simulink model "gm_soc_dvbs2_fpga"  (R2025b)
settings: Solver=VariableStepAuto  StartTime=0.0  StopTime=10.0  RelTol=1e-3
InitFcn:
  | soc_dvbs2_init;
undefined symbols (not defined in the file or in its folder): Add, coefficientsLog, coefficientsSqrt1, coefficientsSqrt2, dataBits, Deinterleaver, designMultirateFIR, noisePow, Shift, Short, soc_dvbs2_designFIRFilter, soc_dvbs2_txPacketBits, syncWord, txDataOut, txFiltCoeff, XData
libraries: simulink x304, hdlsllib x265, dspsigops x15, dsphdlfiltering2 x8, hdlmdlgenlib x6, dsphdlsigops2 x5, commseqgen3 x5, dsphdlmathfun2 x3, hwlogicconnlib x2, whdledac x2, commhdlcrc x2, whdlutilities x1
(part 23 of 36)

== system gm_soc_dvbs2_fpga/DVBS2/DVBS2 TxRx/DVB-S2 HDL Receiver/Synchronizer and PL Header Decoder/Time Frequency and Coarse Phase Synchronizer/Coarse Phase Synchronizer/Coarse Phase Estimator ==
  dataIn : Inport  OutDataTypeStr=fixdt(1, 18, 13)  PortDimensions=1  SampleTime=2.5e-07
      settings: SignalType=complex
  pilotIdx : Inport  Port=2  OutDataTypeStr=fixdt(0, 11, 0)  PortDimensions=1  SampleTime=2.5e-07
  pilotValid : Inport  Port=3  OutDataTypeStr=boolean  PortDimensions=1  SampleTime=2.5e-07
  Add3 : Sum  OutDataTypeStr=fixdt(1, 17, 14)  AccumDataTypeStr=fixdt(1, 18, 14)  SampleTime=2.5e-07
  Compare To Constant1 : simulink/Logic and Bit Operations/Compare To Constant  relop===  const="fi(0,0,11,0,\"hex\",\"5c3\")"  OutDataTypeStr=boolean
  Compare To Constant2 : simulink/Logic and Bit Operations/Compare To Constant  relop===  const="fi(0,0,11,0,\"hex\",\"5a0\")"  OutDataTypeStr=boolean
  Data Type Conversion : DataTypeConversion  OutDataTypeStr=fixdt(1, 17, 14)  SampleTime=2.5e-07  SaturateOnIntegerOverflow=off  RndMeth=Floor
  Delay{,1,8..11,15..17} (9 alike) : Delay  DelayLength=double(1)  InitialCondition=0  SampleTime=2.5e-07
  Delay{2..7,12..14,20} (10 alike) : Delay  DelayLength=double(2)  InitialCondition=0  SampleTime=2.5e-07
  Gain : Gain  Gain="fi(0,1,18,17,\"hex\",\"16a0a + 295f6 i\")"  ParamDataTypeStr=fixdt(1, 18, 17)  OutDataTypeStr=fixdt(1, 18, 13)  SampleTime=2.5e-07
  Gain1 : Gain  Gain="fi(0,0,5,5,\"hex\",\"01\")"  ParamDataTypeStr=fixdt(0, 5, 5)  OutDataTypeStr=fixdt(1, 18, 13)  SampleTime=2.5e-07
  Logical Operator : Logic  AllPortsSameDT=off  OutDataTypeStr=boolean  SampleTime=2.5e-07
  Logical Operator1 : Logic  AllPortsSameDT=off  OutDataTypeStr=boolean  SampleTime=2.5e-07
  Unit Delay Enabled Resettable Synchronous : hdlsllib/Discrete/Unit Delay Enabled Resettable Synchronous  InitialCondition=double(0)  SampleTime=-1
  estimate : Outport  SampleTime=2.5e-07
  estValid : Outport  Port=2  SampleTime=2.5e-07
  wires:
  Delay10/1 -> Unit Delay Enabled Resettable Synchronous/3
  pilotValid/1 -> Delay5/1, Delay16/1, Delay/1
  Delay/1 -> Delay7/1
  dataIn/1 -> Delay1/1
  Delay15/1 -> Compare To Constant1/1
  pilotIdx/1 -> Delay15/1, Compare To Constant2/1
  Delay1/1 -> Delay4/1
  Compare To Constant2/1 -> Delay6/1
  Compare To Constant1/1 -> Delay14/1
  Delay4/1 -> Gain/1
  Delay16/1 -> Delay13/1
  Delay6/1 -> Logical Operator/1
  Delay5/1 -> Logical Operator/2
  Gain/1 -> Delay2/1
  Delay14/1 -> Logical Operator1/1
  Delay13/1 -> Logical Operator1/2
  Delay7/1 -> Delay3/1
  Logical Operator/1 -> Delay20/1
  Delay2/1 -> Gain1/1
  Logical Operator1/1 -> Delay12/1
  Delay3/1 -> Delay9/1
  Delay20/1 -> Delay10/1
  Gain1/1 -> Data Type Conversion/1
  Delay12/1 -> Delay11/1
  Delay9/1 -> Unit Delay Enabled Resettable Synchronous/2
  Data Type Conversion/1 -> Delay8/1
  Delay11/1 -> Delay17/1
  Unit Delay Enabled Resettable Synchronous/1 -> estimate/1, Add3/1
  Delay8/1 -> Add3/2
  Delay17/1 -> estValid/1
  Add3/1 -> Unit Delay Enabled Resettable Synchronous/1

== system gm_soc_dvbs2_fpga/DVBS2/DVBS2 TxRx/DVB-S2 HDL Receiver/Synchronizer and PL Header Decoder/Time Frequency and Coarse Phase Synchronizer/Coarse Phase Synchronizer/Unwrapping algorithm ==
  u : Inport  OutDataTypeStr=fixdt(1, 17, 14)  PortDimensions=1  SampleTime=2.5e-07
      settings: SignalType=complex
  E : Inport  Port=2  OutDataTypeStr=boolean  PortDimensions=1  SampleTime=2.5e-07
  Add : Sum  Inputs=+-  OutDataTypeStr=fixdt(1, 20, 19)  AccumDataTypeStr=fixdt(1, 26, 20)  SampleTime=2.5e-07
  Add1 : Sum  OutDataTypeStr=fixdt(1, 25, 20)  AccumDataTypeStr=fixdt(1, 26, 20)  SampleTime=2.5e-07
  Complex to Magnitude-Angle HDL Optimized : dsphdlmathfun2/Complex to Magnitude-Angle  NumIterationsSource=Auto  NumIterations=10  OutputFormat=Angle  AngleFormat=Normalized  ScaleOutput=on  ScalingMethod=Shift-Add  SimulateUsing=Code generation
  Constant : Constant  OutDataTypeStr=boolean  SampleTime=2.5e-07
  Data Type Conversion : DataTypeConversion  OutDataTypeStr=fixdt(1, 25, 20)  SampleTime=2.5e-07  SaturateOnIntegerOverflow=off  RndMeth=Floor
  Data Type Conversion1 : DataTypeConversion  OutDataTypeStr=fixdt(1, 21, 21)  SampleTime=2.5e-07  SaturateOnIntegerOverflow=off  RndMeth=Floor
  Data Type Conversion2 : DataTypeConversion  OutDataTypeStr=fixdt(1, 21, 0)  ConvertRealWorld=Stored Integer (SI)  SampleTime=2.5e-07  SaturateOnIntegerOverflow=off  RndMeth=Floor
  Gain1 : Gain  Gain="fi(0,0,1,1,\"hex\",\"1\")"  ParamDataTypeStr=fixdt(0, 1, 1)  OutDataTypeStr=fixdt(1, 26, 21)  SampleTime=2.5e-07
  NCO HDL Optimized : dsphdlsigops2/NCO  PhaseIncrementSource=Property  PhaseIncrement=0  PhaseOffsetSource=Input port  PhaseOffset=0  DitherSource=None  NumDitherBits=4  SamplesPerFrame=1  LUTCompress=off  ResetAction=off  Waveform=Complex exponential  PhasePort=off  SimulateUsing=Code generation  AccumulatorWL=21  PhaseQuantization=on  NumQuantizerAccumulatorBits=14  OutputDataType=Binary point scaling  OutputWL=16  OutputFL=14
  NCO HDL Optimized_term1 : Terminator
  PrevEst : hdlsllib/Discrete/Unit Delay Enabled Synchronous  InitialCondition=double(0)  SampleTime=-1
  currentEst : hdlsllib/Discrete/Unit Delay Enabled Synchronous  InitialCondition=double(0)  SampleTime=-1
  estimate : Outport  SampleTime=2.5e-07  VectorParamsAs1DForOutWhenUnconnected=off
  wires:
  u/1 -> Complex to Magnitude-Angle HDL Optimized/1
  E/1 -> Complex to Magnitude-Angle HDL Optimized/2
  Complex to Magnitude-Angle HDL Optimized/1 -> currentEst/1
  Data Type Conversion1/1 -> Data Type Conversion2/1
  currentEst/1 -> Add/1
  Complex to Magnitude-Angle HDL Optimized/2 -> PrevEst/2, currentEst/2
  Data Type Conversion/1 -> Add1/1
  PrevEst/1 -> Add1/2, Add/2
  Add/1 -> Data Type Conversion/1
  Add1/1 -> Gain1/1, PrevEst/1
  Gain1/1 -> Data Type Conversion1/1
  Data Type Conversion2/1 -> NCO HDL Optimized/1
  Constant/1 -> NCO HDL Optimized/2
  NCO HDL Optimized/1 -> estimate/1
  NCO HDL Optimized/2 -> NCO HDL Optimized_term1/1

== system gm_soc_dvbs2_fpga/DVBS2/DVBS2 TxRx/DVB-S2 HDL Receiver/Synchronizer and PL Header Decoder/Time Frequency and Coarse Phase Synchronizer/Fine Frequency Synchronizer/Modified L and R Algorithm ==
  z : Inport  OutDataTypeStr=fixdt(1, 18, 13)  PortDimensions=1  SampleTime=2.5e-07
      settings: SignalType=complex
  zvalid : Inport  Port=2  OutDataTypeStr=boolean  PortDimensions=1  SampleTime=2.5e-07
  pilotIdx : Inport  Port=3  OutDataTypeStr=fixdt(0, 11, 0)  PortDimensions=1  SampleTime=2.5e-07
  Compare To Constant2 : simulink/Logic and Bit Operations/Compare To Constant  relop===  const=config.PilotMaxIdx  OutDataTypeStr=boolean
  Complex to Magnitude-Angle HDL Optimized : dsphdlmathfun2/Complex to Magnitude-Angle  NumIterationsSource=Auto  NumIterations=10  OutputFormat=Angle  AngleFormat=Normalized  ScaleOutput=on  ScalingMethod=Shift-Add  SimulateUsing=Code generation
  Data Type Conversion : DataTypeConversion  OutDataTypeStr=fixdt(1,21,21)  SaturateOnIntegerOverflow=off  RndMeth=Floor
  Data Type Conversion1 : DataTypeConversion  OutDataTypeStr=fixdt(1,43,26)  SaturateOnIntegerOverflow=off  RndMeth=Floor
  Data Type Conversion3 : DataTypeConversion  OutDataTypeStr=fixdt(1,43,40)  ConvertRealWorld=Stored Integer (SI)  SaturateOnIntegerOverflow=off  RndMeth=Floor
  Delay : Delay
  Delay1 : Delay
  Delay2 : Delay
  Delay3 : Delay  DelayLength=28
  Delay4 : Delay  DelayLength=1
  Gain : Gain  Gain=fi(1/19,0,16,16)  ParamDataTypeStr=Inherit: Inherit from 'Gain'  OutDataTypeStr=fixdt(1, 46, 45)
  L and R Algorithm 18 point : Subsystem
  Logical Operator : Logic  AllPortsSameDT=off  OutDataTypeStr=boolean
  Moving Average : Subsystem
  Unit Delay Enabled Synchronous : hdlsllib/Discrete/Unit Delay Enabled Synchronous  InitialCondition=0.0  SampleTime=-1
  estOut : Outport  SampleTime=2.5e-07
  wires:
  Compare To Constant2/1 -> Logical Operator/2
  Logical Operator/1 -> Delay3/1
  L and R Algorithm 18 point/1(dataIn) -> Moving Average/1(dataIn)
  z/1 -> L and R Algorithm 18 point/1(z)
  Complex to Magnitude-Angle HDL Optimized/1 -> Unit Delay Enabled Synchronous/1
  pilotIdx/1 -> Compare To Constant2/1
  Unit Delay Enabled Synchronous/1 -> Delay4/1
  zvalid/1 -> Logical Operator/1, L and R Algorithm 18 point/2(zvalid)
  Delay3/1 -> Delay/1
  Delay/1 -> Moving Average/2(validIn)
  Moving Average/1(dataOut) -> Data Type Conversion1/1
  Moving Average/2(validOut) -> Complex to Magnitude-Angle HDL Optimized/2
  Data Type Conversion1/1 -> Data Type Conversion3/1
  Data Type Conversion3/1 -> Complex to Magnitude-Angle HDL Optimized/1
  Complex to Magnitude-Angle HDL Optimized/2 -> Unit Delay Enabled Synchronous/2
  Delay4/1 -> Delay1/1
  Delay1/1 -> Gain/1
  Gain/1 -> Delay2/1
  Delay2/1 -> Data Type Conversion/1
  Data Type Conversion/1 -> estOut/1

== system gm_soc_dvbs2_fpga/DVBS2/DVBS2 TxRx/DVB-S2 HDL Receiver/Synchronizer and PL Header Decoder/Time Frequency and Coarse Phase Synchronizer/Fine Gain Control/Reciprocal ==
  dataIn : Inport  OutDataTypeStr=fixdt(1, 13, 10)  PortDimensions=1  SampleTime=2.5e-07
  Compare To Constant : simulink/Logic and Bit Operations/Compare To Constant  relop=<  const=0  OutDataTypeStr=boolean
  Compare To Constant1 : simulink/Logic and Bit Operations/Compare To Constant  relop===  const=0  OutDataTypeStr=boolean
  Constant : Constant  OutDataTypeStr=fixdt(1, 26, 14)  SampleTime=-1
  Data Type Conversion : DataTypeConversion  OutDataTypeStr=fixdt(1,WL,0)  ConvertRealWorld=Stored Integer (SI)  SaturateOnIntegerOverflow=off  RndMeth=Floor
  Data Type Conversion1 : DataTypeConversion  OutDataTypeStr=fixdt(0,LUTAddrWL,0)  ConvertRealWorld=Stored Integer (SI)  SaturateOnIntegerOverflow=off  RndMeth=Floor
      mask init:
      | Simulink.suppressDiagnostic(gcb, 'SimulinkFixedPoint:util:Overflowoccurred');
  Data Type Conversion2 : DataTypeConversion  OutDataTypeStr=fixdt(0,WL-LUTAddrWL,0)  ConvertRealWorld=Stored Integer (SI)  SaturateOnIntegerOverflow=off  RndMeth=Floor
  Delay : Delay  DelayLength=1
  Delay1 : Delay  DelayLength=1
  Delay2 : Delay  DelayLength=1
  Delay3 : Delay  DelayLength=7
  Extract Bits : simulink/Logic and Bit Operations/Extract Bits  bitsToExtract=Range ending with least significant bit  numBits=LUTAddrWL  bitIdxRange=[0 7]  outScalingMode=Treat bit field as an integer
  Function Impl : Subsystem
  Switch : Switch  Criteria=u2 > Threshold  OutDataTypeStr=fixdt(1, 26, 14)  SaturateOnIntegerOverflow=off  InputSameDT=off
  dataOut : Outport  SampleTime=2.5e-07
  wires:
  dataIn/1 -> Data Type Conversion/1, Delay3/1
  Delay1/1 -> Data Type Conversion2/1
  Delay3/1 -> Compare To Constant1/1
  Compare To Constant1/1 -> Switch/2
  Data Type Conversion/1 -> Delay/1
  Compare To Constant/1 -> Delay1/1
  Delay/1 -> Extract Bits/1, Compare To Constant/1
  Extract Bits/1 -> Delay2/1
  Delay2/1 -> Data Type Conversion1/1
  Data Type Conversion2/1 -> Function Impl/1(switch)
  Data Type Conversion1/1 -> Function Impl/2(LUTAddr)
  Constant/1 -> Switch/1
  Function Impl/1(functionValues) -> Switch/3
  Switch/1 -> dataOut/1

== system gm_soc_dvbs2_fpga/DVBS2/DVBS2 TxRx/DVB-S2 HDL Receiver/Synchronizer and PL Header Decoder/Time Frequency and Coarse Phase Synchronizer/Time and Coarse Frequency Synchronizer/Coarse Frequency Estimator ==
  rst : Inport  OutDataTypeStr=boolean  PortDimensions=1  SampleTime=2.5e-07
  dataIn : Inport  Port=2  OutDataTypeStr=fixdt(1, 18, 13)  PortDimensions=1  SampleTime=2.5e-07
      settings: SignalType=complex
  pilotValid : Inport  Port=3  OutDataTypeStr=boolean  PortDimensions=1  SampleTime=2.5e-07
  pilotIdx : Inport  Port=4  OutDataTypeStr=fixdt(0, 11, 0)  PortDimensions=1  SampleTime=2.5e-07
  Compare To Constant : simulink/Logic and Bit Operations/Compare To Constant  relop=>  const="fi(0,0,16,0,\"hex\",\"0020\")"  OutDataTypeStr=boolean
  Constant : Constant  Value=0  OutDataTypeStr=boolean  SampleTime=6.25e-08
  Delay : Delay  DelayLength=double(1)  InitialCondition=1  SampleTime=6.25e-08
  Delay{1..4,28} (5 alike) : Delay  DelayLength=double(1)  InitialCondition=0  SampleTime=2.5e-07
  Direct Digital Synthesis : Subsystem
  Frequency Error Detector : Subsystem
  Logical Operator : Logic  Operator=NOT  Inputs=1  AllPortsSameDT=off  OutDataTypeStr=boolean  SampleTime=2.5e-07
  Loop Filter : Subsystem
  Multiport Switch : MultiPortSwitch  DataPortOrder=Zero-based contiguous  Inputs=2  DiagnosticForDefault=None  zeroidx=on  OutDataTypeStr=fixdt(1, 16, 14)  SampleTime=6.25e-08  SaturateOnIntegerOverflow=off  InputSameDT=off
  Pilot Blks Counter : Subsystem
  Unit Delay Enabled Resettable Synchronous : hdlsllib/Discrete/Unit Delay Enabled Resettable Synchronous  InitialCondition=double(0)  SampleTime=-1
  complexEstimate : Outport  SampleTime=6.25e-08
  normFreqEst : Outport  Port=2  SampleTime=2.5e-07
  wires:
  pilotIdx/1 -> Pilot Blks Counter/1(pilotIdx), Frequency Error Detector/2(pilotIdx)
  dataIn/1 -> Frequency Error Detector/1(dataIn)
  Delay2/1 -> Loop Filter/2(rst)
  rst/1 -> Unit Delay Enabled Resettable Synchronous/3, Delay2/1, Pilot Blks Counter/3(rst)
  pilotValid/1 -> Frequency Error Detector/3(pilotValid), Pilot Blks Counter/2(pilotValid)
  Pilot Blks Counter/1(pilotBlkCount) -> Compare To Constant/1
  Frequency Error Detector/1(e) -> Delay28/1
  Compare To Constant/1 -> Unit Delay Enabled Resettable Synchronous/2, Unit Delay Enabled Resettable Synchronous/1
  Delay28/1 -> Loop Filter/1(e)
  Loop Filter/2(rstOut) -> Delay4/1
  Unit Delay Enabled Resettable Synchronous/1 -> Logical Operator/1
  Logical Operator/1 -> Delay1/1
  Delay1/1 -> Loop Filter/3(En)
  Loop Filter/1(v) -> Delay3/1
  Delay3/1 -> Direct Digital Synthesis/1(v)
  Delay4/1 -> Direct Digital Synthesis/2(rst)
  Constant/1 -> Multiport Switch/1
  Direct Digital Synthesis/1(complexEst) -> Multiport Switch/3
  Direct Digital Synthesis/2(normalizedEst) -> normFreqEst/1
  Multiport Switch/1 -> complexEstimate/1, Delay/1
  Delay/1 -> Multiport Switch/2

== system gm_soc_dvbs2_fpga/DVBS2/DVBS2 TxRx/DVB-S2 HDL Receiver/Synchronizer and PL Header Decoder/Time Frequency and Coarse Phase Synchronizer/Time and Coarse Frequency Synchronizer/Frame Synchronizer ==
  dataIn : Inport  OutDataTypeStr=fixdt(1, 18, 13)  PortDimensions=1  SampleTime=2.5e-07
      settings: SignalType=complex
  validIn : Inport  Port=2  OutDataTypeStr=boolean  PortDimensions=1  SampleTime=2.5e-07
  Correlator : Subsystem
  Data Type Conversion : DataTypeConversion  OutDataTypeStr=fixdt(1,15,12)  SaturateOnIntegerOverflow=off  RndMeth=Floor
  Data Type Conversion1 : DataTypeConversion  OutDataTypeStr=fixdt(1,15,11)  SaturateOnIntegerOverflow=off  RndMeth=Floor
  Data Type Conversion2 : DataTypeConversion  OutDataTypeStr=fixdt(1,15,12)  SaturateOnIntegerOverflow=off  RndMeth=Floor
  Delay1 : Delay  DelayLength=70
  Delay{6,9..11} (4 alike) : Delay  DelayLength=9
  Delay12 : Delay
  Delay13 : Delay
  Delay2 : Delay  DelayLength=70
  Delay3 : Delay  DelayLength=config.PLSCLength
  Delay4 : Delay  DelayLength=config.PLSCLength
  Delay5 : Delay  DelayLength=config.PLSCLength
  Pilot and Sync Pulse Indicator : Subsystem
  dataOut : Outport  SampleTime=2.5e-07
  validOut : Outport  Port=2  SampleTime=2.5e-07
  endOfSOF : Outport  Port=3  SampleTime=2.5e-07
  hasPilots : Outport  Port=4  SampleTime=2.5e-07
  VisualizeCorrelationSignals : Outport  Port=5
  wires:
  Pilot and Sync Pulse Indicator/1(hasPilots) -> hasPilots/1
  Delay6/1 -> Delay1/1
  Data Type Conversion/1 -> Pilot and Sync Pulse Indicator/1(SOFCorrDelayed)
  dataIn/1 -> Delay12/1
  validIn/1 -> Delay13/1
  Delay12/1 -> Delay6/1, Correlator/1(dataIn)
  Delay13/1 -> Delay11/1, Correlator/2(validIn)
  Correlator/1(SOFCorrOut) -> Delay5/1
  Correlator/2(PLSCCorrOut) -> Data Type Conversion1/1
  Correlator/3(threshold) -> Data Type Conversion2/1
  Delay11/1 -> Delay2/1
  Delay1/1 -> Delay3/1
  Delay5/1 -> Data Type Conversion/1
  Data Type Conversion2/1 -> Pilot and Sync Pulse Indicator/3(threshold)
  Delay2/1 -> Delay4/1
  Delay3/1 -> Delay10/1
  Data Type Conversion1/1 -> Pilot and Sync Pulse Indicator/2(PLSCCorr)
  Delay4/1 -> Delay9/1
  Delay10/1 -> dataOut/1
  Pilot and Sync Pulse Indicator/2(thresholdExceeded) -> endOfSOF/1
  Pilot and Sync Pulse Indicator/3(VisualizeCorrelationSignals) -> VisualizeCorrelationSignals/1
  Delay9/1 -> validOut/1

== system gm_soc_dvbs2_fpga/DVBS2/DVBS2 TxRx/DVB-S2 HDL Receiver/Synchronizer and PL Header Decoder/Time Frequency and Coarse Phase Synchronizer/Time and Coarse Frequency Synchronizer/PL Data Descrambler and Pilot Valid Indicator ==
  dataIn : Inport  OutDataTypeStr=fixdt(1, 18, 13)  PortDimensions=1  SampleTime=2.5e-07
      settings: SignalType=complex
  validIn : Inport  Port=2  OutDataTypeStr=boolean  PortDimensions=1  SampleTime=2.5e-07
  endOfSOFIn : Inport  Port=3  OutDataTypeStr=boolean  PortDimensions=1  SampleTime=2.5e-07
  hasPilots : Inport  Port=4  OutDataTypeStr=boolean  PortDimensions=1  SampleTime=2.5e-07
  Compare To Constant1 : simulink/Logic and Bit Operations/Compare To Constant  relop===  const=config.PLSCLength - 1  OutDataTypeStr=boolean
  Delay : Delay  DelayLength=config.SOFLength
  Delay1 : Delay  DelayLength=config.SOFLength
  Delay{2..18} (17 alike) : Delay  DelayLength=1
  Delay{19..22} (4 alike) : Delay  DelayLength=14
  Delay23 : Delay  DelayLength=4
  Delay24 : Delay  DelayLength=4
  Input Sample Counter : hdlsllib/Sources/HDL Counter  CountType=Free running  CountInit=0  CountStep=1  CountMax=25  CountFromType=Initial value  CountFrom=0  CountResetPort=on  CountLoadPort=off  CountEnbPort=on  CountDirPort=off  CountHitOutputPort=off  CountDataType=Unsigned  CountWordLen=32  CountFracLen=0  CountSampTime=1
  Logical Operator : Logic  AllPortsSameDT=off  OutDataTypeStr=boolean
  PL Data Descrambler : Subsystem
  Pilot Valid Indicator : Subsystem
  pilotidx : Outport  SampleTime=2.5e-07
  pilotValid : Outport  Port=2  SampleTime=2.5e-07
  dataOut : Outport  Port=3  SampleTime=2.5e-07
  validOut : Outport  Port=4  SampleTime=2.5e-07
  endOfSOF : Outport  Port=5  SampleTime=2.5e-07
  wires:
  endOfSOFIn/1 -> Delay2/1
  validIn/1 -> Delay9/1
  Delay2/1 -> Delay5/1, Input Sample Counter/1
  Delay9/1 -> Input Sample Counter/2, Delay7/1
  hasPilots/1 -> Delay3/1
  Input Sample Counter/1 -> Delay6/1
  Delay7/1 -> Delay12/1, [validIn]
  Delay5/1 -> Delay16/1
  Delay6/1 -> Delay13/1, Compare To Constant1/1
  dataIn/1 -> Delay10/1
  Delay3/1 -> Delay4/1
  Delay/1 -> Delay23/1
  Delay16/1 -> Delay20/1
  [validIn] -> Delay15/1
  Compare To Constant1/1 -> Delay14/1
  Delay10/1 -> Delay8/1
  Delay4/1 -> Delay18/1
  [validIn] -> Delay17/1
  PL Data Descrambler/1(dataOut) -> Delay/1
  Delay15/1 -> Logical Operator/1
  Pilot Valid Indicator/2(pilotIdx) -> pilotidx/1
  Delay14/1 -> Logical Operator/2
  Delay20/1 -> Pilot Valid Indicator/3(endOfSOFIn)
  Delay13/1 -> PL Data Descrambler/2(inputCount)
  Delay8/1 -> Delay11/1
  Delay18/1 -> Delay22/1
  Delay1/1 -> Delay24/1
  Delay17/1 -> Delay21/1
  Logical Operator/1 -> Delay19/1, PL Data Descrambler/1(reset)
  Delay12/1 -> PL Data Descrambler/3(validIn)
  Pilot Valid Indicator/1(pilotValid) -> pilotValid/1
  Delay11/1 -> PL Data Descrambler/4(dataIn)
  Delay22/1 -> Pilot Valid Indicator/1(pilotEnable)
  Delay21/1 -> Pilot Valid Indicator/2(validIn)
  Delay19/1 -> Pilot Valid Indicator/4(endOfPLSC)
  PL Data Descrambler/2(validOut) -> Delay1/1
  Pilot Valid Indicator/3(endOfSOF) -> endOfSOF/1
  Delay23/1 -> dataOut/1
  Delay24/1 -> validOut/1

== system gm_soc_dvbs2_fpga/DVBS2/DVBS2 TxRx/DVB-S2 HDL Receiver/Synchronizer and PL Header Decoder/Time Frequency and Coarse Phase Synchronizer/Time and Coarse Frequency Synchronizer/Symbol Synchronizer ==
  dataIn : Inport  OutDataTypeStr=fixdt(1, 18, 13)  PortDimensions=1  SampleTime=6.25e-08
      settings: SignalType=complex
  validIn : Inport  Port=2  OutDataTypeStr=boolean  PortDimensions=1  SampleTime=6.25e-08
  Data Type Conversion : DataTypeConversion  OutDataTypeStr=fixdt(1, 18, 13)  SampleTime=6.25e-08  SaturateOnIntegerOverflow=off  RndMeth=Floor
  Delay{1..4,6,8..9} (7 alike) : Delay  DelayLength=double(1)  InitialCondition=0  SampleTime=6.25e-08
  Delay5 : Delay  DelayLength=double(12)  InitialCondition=0  SampleTime=6.25e-08
  Delay7 : Delay  DelayLength=double(12)  InitialCondition=0  SampleTime=6.25e-08
  Gardner TED : Subsystem
  Integer Delay{1..4} (4 alike) : Delay  DelayLength=double(1)  InitialCondition=0  SampleTime=6.25e-08
  Interpolation Control : Subsystem
  Interpolation Filter : Subsystem
  Loop Filter : Subsystem
  Rate Handle : Subsystem
  dataOut : Outport  SampleTime=2.5e-07
  validOut : Outport  Port=2  SampleTime=2.5e-07
  wires:
  Loop Filter/1(v) -> Delay4/1
  Interpolation Control/2(Underflow) -> Integer Delay3/1
  Delay4/1 -> Interpolation Control/1(Delta)
  dataIn/1 -> Integer Delay1/1
  Delay5/1 -> Delay2/1, Delay9/1
  Interpolation Control/1(mu) -> Integer Delay4/1
  Integer Delay3/1 -> Delay5/1
  Integer Delay4/1 -> Interpolation Filter/2(mu)
  Gardner TED/1(e) -> Delay3/1
  Integer Delay1/1 -> Interpolation Filter/1(In)
  validIn/1 -> Integer Delay2/1
  Delay1/1 -> Rate Handle/1(dataIn)
  Interpolation Filter/1(interpolant) -> Delay8/1, Data Type Conversion/1
  Integer Delay2/1 -> Delay7/1
  Delay8/1 -> Gardner TED/1(data)
  Delay9/1 -> Gardner TED/2(strobe)
  Data Type Conversion/1 -> Delay1/1
  Delay7/1 -> Delay6/1
  Delay2/1 -> Rate Handle/2(strobe)
  Delay6/1 -> Rate Handle/3(validIn)
  Delay3/1 -> Loop Filter/1(e)
  Rate Handle/1(dataOut) -> dataOut/1
  Rate Handle/2(validOut) -> validOut/1

== system gm_soc_dvbs2_fpga/DVBS2/DVBS2 TxRx/LUT Based Tx/Subsystem1/Subsystem/txLUT1/1-D Lookup Table ==
  In1 : Inport
  1-D Lookup Table : Lookup_n-D  NumberOfTableDimensions=1  BreakpointsSpecification=Even spacing  BreakpointsForDimension1=0:length(txDataOut)-1  BreakpointsForDimension1FirstPoint=0  Table=fi(DataLUT,1,18,16)  TableDataTypeStr=Inherit: Inherit from 'Table data'  InterpMethod=Flat  InternalRulePriority=Speed  OutDataTypeStr=fixdt(1, 18, 16)  RndMeth=Simplest
  1-D Lookup Table_pd1 : Delay  DelayLength=1
  Out1 : Outport
  wires:
  In1/1 -> 1-D Lookup Table/1
  1-D Lookup Table_pd1/1 -> Out1/1
  1-D Lookup Table/1 -> 1-D Lookup Table_pd1/1

== system gm_soc_dvbs2_fpga/DVBS2/DVBS2 TxRx/LUT Based Tx/Subsystem1/Subsystem/txLUT2/1-D Lookup Table ==
  In1 : Inport
  1-D Lookup Table : Lookup_n-D  NumberOfTableDimensions=1  BreakpointsSpecification=Even spacing  BreakpointsForDimension1=0:length(txDataOut)-1  BreakpointsForDimension1FirstPoint=0  Table=fi(DataLUT,1,18,16)  TableDataTypeStr=Inherit: Inherit from 'Table data'  InterpMethod=Flat  InternalRulePriority=Speed  OutDataTypeStr=fixdt(1, 18, 16)  RndMeth=Simplest
  1-D Lookup Table_pd1 : Delay  DelayLength=1
  Out1 : Outport
  wires:
  In1/1 -> 1-D Lookup Table/1
  1-D Lookup Table_pd1/1 -> Out1/1
  1-D Lookup Table/1 -> 1-D Lookup Table_pd1/1

== system gm_soc_dvbs2_fpga/DVBS2/DVBS2 TxRx/LUT Based Tx/Subsystem1/Subsystem/txLUT3/1-D Lookup Table ==
  In1 : Inport
  1-D Lookup Table : Lookup_n-D  NumberOfTableDimensions=1  BreakpointsSpecification=Even spacing  BreakpointsForDimension1=0:length(txDataOut)-1  BreakpointsForDimension1FirstPoint=0  Table=fi(DataLUT,1,18,16)  TableDataTypeStr=Inherit: Inherit from 'Table data'  InterpMethod=Flat  InternalRulePriority=Speed  OutDataTypeStr=fixdt(1, 18, 16)  RndMeth=Simplest
  1-D Lookup Table_pd1 : Delay  DelayLength=1
  Out1 : Outport
  wires:
  In1/1 -> 1-D Lookup Table/1
  1-D Lookup Table_pd1/1 -> Out1/1
  1-D Lookup Table/1 -> 1-D Lookup Table_pd1/1

== system gm_soc_dvbs2_fpga/DVBS2/DVBS2 TxRx/LUT Based Tx/Subsystem1/Subsystem/txLUT4/1-D Lookup Table ==
  In1 : Inport
  1-D Lookup Table : Lookup_n-D  NumberOfTableDimensions=1  BreakpointsSpecification=Even spacing  BreakpointsForDimension1=0:length(txDataOut)-1  BreakpointsForDimension1FirstPoint=0  Table=fi(DataLUT,1,18,16)  TableDataTypeStr=Inherit: Inherit from 'Table data'  InterpMethod=Flat  InternalRulePriority=Speed  OutDataTypeStr=fixdt(1, 18, 16)  RndMeth=Simplest
  1-D Lookup Table_pd1 : Delay  DelayLength=1
  Out1 : Outport
  wires:
  In1/1 -> 1-D Lookup Table/1
  1-D Lookup Table_pd1/1 -> Out1/1
  1-D Lookup Table/1 -> 1-D Lookup Table_pd1/1

== system gm_soc_dvbs2_fpga/DVBS2/DVBS2 TxRx/LUT Based Tx/Subsystem1/Subsystem/txLUT5/1-D Lookup Table ==
  In1 : Inport
  1-D Lookup Table : Lookup_n-D  NumberOfTableDimensions=1  BreakpointsSpecification=Even spacing  BreakpointsForDimension1=0:length(txDataOut)-1  BreakpointsForDimension1FirstPoint=0  Table=fi(DataLUT,1,18,16)  TableDataTypeStr=Inherit: Inherit from 'Table data'  InterpMethod=Flat  InternalRulePriority=Speed  OutDataTypeStr=fixdt(1, 18, 16)  RndMeth=Simplest
  1-D Lookup Table_pd1 : Delay  DelayLength=1
  Out1 : Outport
  wires:
  In1/1 -> 1-D Lookup Table/1
  1-D Lookup Table_pd1/1 -> Out1/1
  1-D Lookup Table/1 -> 1-D Lookup Table_pd1/1

== system gm_soc_dvbs2_fpga/DVBS2/DVBS2 TxRx/LUT Based Tx/Subsystem1/Subsystem/txLUT6/1-D Lookup Table ==
  In1 : Inport
  1-D Lookup Table : Lookup_n-D  NumberOfTableDimensions=1  BreakpointsSpecification=Even spacing  BreakpointsForDimension1=0:length(txDataOut)-1  BreakpointsForDimension1FirstPoint=0  Table=fi(DataLUT,1,18,16)  TableDataTypeStr=Inherit: Inherit from 'Table data'  InterpMethod=Flat  InternalRulePriority=Speed  OutDataTypeStr=fixdt(1, 18, 16)  RndMeth=Simplest
  1-D Lookup Table_pd1 : Delay  DelayLength=1
  Out1 : Outport
  wires:
  In1/1 -> 1-D Lookup Table/1
  1-D Lookup Table_pd1/1 -> Out1/1
  1-D Lookup Table/1 -> 1-D Lookup Table_pd1/1

== system gm_soc_dvbs2_fpga/DVBS2/DVBS2 TxRx/LUT Based Tx/Subsystem1/Subsystem1/txLUT1/1-D Lookup Table ==
  In1 : Inport
  1-D Lookup Table : Lookup_n-D  NumberOfTableDimensions=1  BreakpointsSpecification=Even spacing  BreakpointsForDimension1=0:length(txDataOut)-1  BreakpointsForDimension1FirstPoint=0  Table=fi(DataLUT,1,18,16)  TableDataTypeStr=Inherit: Inherit from 'Table data'  InterpMethod=Flat  InternalRulePriority=Speed  OutDataTypeStr=fixdt(1, 18, 16)  RndMeth=Simplest
  1-D Lookup Table_pd1 : Delay  DelayLength=1
  Out1 : Outport
  wires:
  In1/1 -> 1-D Lookup Table/1
  1-D Lookup Table_pd1/1 -> Out1/1
  1-D Lookup Table/1 -> 1-D Lookup Table_pd1/1

== system gm_soc_dvbs2_fpga/DVBS2/DVBS2 TxRx/LUT Based Tx/Subsystem1/Subsystem1/txLUT2/1-D Lookup Table ==
  In1 : Inport
  1-D Lookup Table : Lookup_n-D  NumberOfTableDimensions=1  BreakpointsSpecification=Even spacing  BreakpointsForDimension1=0:length(txDataOut)-1  BreakpointsForDimension1FirstPoint=0  Table=fi(DataLUT,1,18,16)  TableDataTypeStr=Inherit: Inherit from 'Table data'  InterpMethod=Flat  InternalRulePriority=Speed  OutDataTypeStr=fixdt(1, 18, 16)  RndMeth=Simplest
  1-D Lookup Table_pd1 : Delay  DelayLength=1
  Out1 : Outport
  wires:
  In1/1 -> 1-D Lookup Table/1
  1-D Lookup Table_pd1/1 -> Out1/1
  1-D Lookup Table/1 -> 1-D Lookup Table_pd1/1

== system gm_soc_dvbs2_fpga/DVBS2/DVBS2 TxRx/LUT Based Tx/Subsystem1/Subsystem1/txLUT3/1-D Lookup Table ==
  In1 : Inport
  1-D Lookup Table : Lookup_n-D  NumberOfTableDimensions=1  BreakpointsSpecification=Even spacing  BreakpointsForDimension1=0:length(txDataOut)-1  BreakpointsForDimension1FirstPoint=0  Table=fi(DataLUT,1,18,16)  TableDataTypeStr=Inherit: Inherit from 'Table data'  InterpMethod=Flat  InternalRulePriority=Speed  OutDataTypeStr=fixdt(1, 18, 16)  RndMeth=Simplest
  1-D Lookup Table_pd1 : Delay  DelayLength=1
  Out1 : Outport
  wires:
  In1/1 -> 1-D Lookup Table/1
  1-D Lookup Table_pd1/1 -> Out1/1
  1-D Lookup Table/1 -> 1-D Lookup Table_pd1/1

== system gm_soc_dvbs2_fpga/DVBS2/DVBS2 TxRx/LUT Based Tx/Subsystem1/Subsystem1/txLUT4/1-D Lookup Table ==
  In1 : Inport
  1-D Lookup Table : Lookup_n-D  NumberOfTableDimensions=1  BreakpointsSpecification=Even spacing  BreakpointsForDimension1=0:length(txDataOut)-1  BreakpointsForDimension1FirstPoint=0  Table=fi(DataLUT,1,18,16)  TableDataTypeStr=Inherit: Inherit from 'Table data'  InterpMethod=Flat  InternalRulePriority=Speed  OutDataTypeStr=fixdt(1, 18, 16)  RndMeth=Simplest
  1-D Lookup Table_pd1 : Delay  DelayLength=1
  Out1 : Outport
  wires:
  In1/1 -> 1-D Lookup Table/1
  1-D Lookup Table_pd1/1 -> Out1/1
  1-D Lookup Table/1 -> 1-D Lookup Table_pd1/1

== system gm_soc_dvbs2_fpga/DVBS2/DVBS2 TxRx/LUT Based Tx/Subsystem1/Subsystem1/txLUT5/1-D Lookup Table ==
  In1 : Inport
  1-D Lookup Table : Lookup_n-D  NumberOfTableDimensions=1  BreakpointsSpecification=Even spacing  BreakpointsForDimension1=0:length(txDataOut)-1  BreakpointsForDimension1FirstPoint=0  Table=fi(DataLUT,1,18,16)  TableDataTypeStr=Inherit: Inherit from 'Table data'  InterpMethod=Flat  InternalRulePriority=Speed  OutDataTypeStr=fixdt(1, 18, 16)  RndMeth=Simplest
  1-D Lookup Table_pd1 : Delay  DelayLength=1
  Out1 : Outport
  wires:
  In1/1 -> 1-D Lookup Table/1
  1-D Lookup Table_pd1/1 -> Out1/1
  1-D Lookup Table/1 -> 1-D Lookup Table_pd1/1

== system gm_soc_dvbs2_fpga/DVBS2/DVBS2 TxRx/LUT Based Tx/Subsystem1/Subsystem1/txLUT6/1-D Lookup Table ==
  In1 : Inport
  1-D Lookup Table : Lookup_n-D  NumberOfTableDimensions=1  BreakpointsSpecification=Even spacing  BreakpointsForDimension1=0:length(txDataOut)-1  BreakpointsForDimension1FirstPoint=0  Table=fi(DataLUT,1,18,16)  TableDataTypeStr=Inherit: Inherit from 'Table data'  InterpMethod=Flat  InternalRulePriority=Speed  OutDataTypeStr=fixdt(1, 18, 16)  RndMeth=Simplest
  1-D Lookup Table_pd1 : Delay  DelayLength=1
  Out1 : Outport
  wires:
  In1/1 -> 1-D Lookup Table/1
  1-D Lookup Table_pd1/1 -> Out1/1
  1-D Lookup Table/1 -> 1-D Lookup Table_pd1/1

== system gm_soc_dvbs2_fpga/DVBS2/DVBS2 TxRx/LUT Based Tx/Subsystem1/Subsystem2/txLUT1/1-D Lookup Table ==
  In1 : Inport
  1-D Lookup Table : Lookup_n-D  NumberOfTableDimensions=1  BreakpointsSpecification=Even spacing  BreakpointsForDimension1=0:length(txDataOut)-1  BreakpointsForDimension1FirstPoint=0  Table=fi(DataLUT,1,18,16)  TableDataTypeStr=Inherit: Inherit from 'Table data'  InterpMethod=Flat  InternalRulePriority=Speed  OutDataTypeStr=fixdt(1, 18, 16)  RndMeth=Simplest
  1-D Lookup Table_pd1 : Delay  DelayLength=1
  Out1 : Outport
  wires:
  In1/1 -> 1-D Lookup Table/1
  1-D Lookup Table_pd1/1 -> Out1/1
  1-D Lookup Table/1 -> 1-D Lookup Table_pd1/1

== system gm_soc_dvbs2_fpga/DVBS2/DVBS2 TxRx/LUT Based Tx/Subsystem1/Subsystem2/txLUT2/1-D Lookup Table ==
  In1 : Inport
  1-D Lookup Table : Lookup_n-D  NumberOfTableDimensions=1  BreakpointsSpecification=Even spacing  BreakpointsForDimension1=0:length(txDataOut)-1  BreakpointsForDimension1FirstPoint=0  Table=fi(DataLUT,1,18,16)  TableDataTypeStr=Inherit: Inherit from 'Table data'  InterpMethod=Flat  InternalRulePriority=Speed  OutDataTypeStr=fixdt(1, 18, 16)  RndMeth=Simplest
  1-D Lookup Table_pd1 : Delay  DelayLength=1
  Out1 : Outport
  wires:
  In1/1 -> 1-D Lookup Table/1
  1-D Lookup Table_pd1/1 -> Out1/1
  1-D Lookup Table/1 -> 1-D Lookup Table_pd1/1

== system gm_soc_dvbs2_fpga/DVBS2/DVBS2 TxRx/LUT Based Tx/Subsystem1/Subsystem2/txLUT3/1-D Lookup Table ==
  In1 : Inport
  1-D Lookup Table : Lookup_n-D  NumberOfTableDimensions=1  BreakpointsSpecification=Even spacing  BreakpointsForDimension1=0:length(txDataOut)-1  BreakpointsForDimension1FirstPoint=0  Table=fi(DataLUT,1,18,16)  TableDataTypeStr=Inherit: Inherit from 'Table data'  InterpMethod=Flat  InternalRulePriority=Speed  OutDataTypeStr=fixdt(1, 18, 16)  RndMeth=Simplest
  1-D Lookup Table_pd1 : Delay  DelayLength=1
  Out1 : Outport
  wires:
  In1/1 -> 1-D Lookup Table/1
  1-D Lookup Table_pd1/1 -> Out1/1
  1-D Lookup Table/1 -> 1-D Lookup Table_pd1/1

== system gm_soc_dvbs2_fpga/DVBS2/DVBS2 TxRx/LUT Based Tx/Subsystem1/Subsystem2/txLUT4/1-D Lookup Table ==
  In1 : Inport
  1-D Lookup Table : Lookup_n-D  NumberOfTableDimensions=1  BreakpointsSpecification=Even spacing  BreakpointsForDimension1=0:length(txDataOut)-1  BreakpointsForDimension1FirstPoint=0  Table=fi(DataLUT,1,18,16)  TableDataTypeStr=Inherit: Inherit from 'Table data'  InterpMethod=Flat  InternalRulePriority=Speed  OutDataTypeStr=fixdt(1, 18, 16)  RndMeth=Simplest
  1-D Lookup Table_pd1 : Delay  DelayLength=1
  Out1 : Outport
  wires:
  In1/1 -> 1-D Lookup Table/1
  1-D Lookup Table_pd1/1 -> Out1/1
  1-D Lookup Table/1 -> 1-D Lookup Table_pd1/1

== system gm_soc_dvbs2_fpga/DVBS2/DVBS2 TxRx/LUT Based Tx/Subsystem1/Subsystem2/txLUT5/1-D Lookup Table ==
  In1 : Inport
  1-D Lookup Table : Lookup_n-D  NumberOfTableDimensions=1  BreakpointsSpecification=Even spacing  BreakpointsForDimension1=0:length(txDataOut)-1  BreakpointsForDimension1FirstPoint=0  Table=fi(DataLUT,1,18,16)  TableDataTypeStr=Inherit: Inherit from 'Table data'  InterpMethod=Flat  InternalRulePriority=Speed  OutDataTypeStr=fixdt(1, 18, 16)  RndMeth=Simplest
  1-D Lookup Table_pd1 : Delay  DelayLength=1
  Out1 : Outport
  wires:
  In1/1 -> 1-D Lookup Table/1
  1-D Lookup Table_pd1/1 -> Out1/1
  1-D Lookup Table/1 -> 1-D Lookup Table_pd1/1

== system gm_soc_dvbs2_fpga/DVBS2/DVBS2 TxRx/LUT Based Tx/Subsystem1/Subsystem2/txLUT6/1-D Lookup Table ==
  In1 : Inport
  1-D Lookup Table : Lookup_n-D  NumberOfTableDimensions=1  BreakpointsSpecification=Even spacing  BreakpointsForDimension1=0:length(txDataOut)-1  BreakpointsForDimension1FirstPoint=0  Table=fi(DataLUT,1,18,16)  TableDataTypeStr=Inherit: Inherit from 'Table data'  InterpMethod=Flat  InternalRulePriority=Speed  OutDataTypeStr=fixdt(1, 18, 16)  RndMeth=Simplest
  1-D Lookup Table_pd1 : Delay  DelayLength=1
  Out1 : Outport
  wires:
  In1/1 -> 1-D Lookup Table/1
  1-D Lookup Table_pd1/1 -> Out1/1
  1-D Lookup Table/1 -> 1-D Lookup Table_pd1/1

== system gm_soc_dvbs2_fpga/DVBS2/DVBS2 TxRx/LUT Based Tx/Subsystem1/Subsystem4/txLUT1/1-D Lookup Table ==
  In1 : Inport
  1-D Lookup Table : Lookup_n-D  NumberOfTableDimensions=1  BreakpointsSpecification=Even spacing  BreakpointsForDimension1=0:length(txDataOut)-1  BreakpointsForDimension1FirstPoint=0  Table=fi(DataLUT,1,18,16)  TableDataTypeStr=Inherit: Inherit from 'Table data'  InterpMethod=Flat  InternalRulePriority=Speed  OutDataTypeStr=fixdt(1, 18, 16)  RndMeth=Simplest
  1-D Lookup Table_pd1 : Delay  DelayLength=1
  Out1 : Outport
  wires:
  In1/1 -> 1-D Lookup Table/1
  1-D Lookup Table/1 -> 1-D Lookup Table_pd1/1
  1-D Lookup Table_pd1/1 -> Out1/1

== system gm_soc_dvbs2_fpga/DVBS2/DVBS2 TxRx/LUT Based Tx/Subsystem1/Subsystem4/txLUT2/1-D Lookup Table ==
  In1 : Inport
  1-D Lookup Table : Lookup_n-D  NumberOfTableDimensions=1  BreakpointsSpecification=Even spacing  BreakpointsForDimension1=0:length(txDataOut)-1  BreakpointsForDimension1FirstPoint=0  Table=fi(DataLUT,1,18,16)  TableDataTypeStr=Inherit: Inherit from 'Table data'  InterpMethod=Flat  InternalRulePriority=Speed  OutDataTypeStr=fixdt(1, 18, 16)  RndMeth=Simplest
  1-D Lookup Table_pd1 : Delay  DelayLength=1
  Out1 : Outport
  wires:
  In1/1 -> 1-D Lookup Table/1
  1-D Lookup Table_pd1/1 -> Out1/1
  1-D Lookup Table/1 -> 1-D Lookup Table_pd1/1

== system gm_soc_dvbs2_fpga/DVBS2/DVBS2 TxRx/LUT Based Tx/Subsystem1/Subsystem4/txLUT3/1-D Lookup Table ==
  In1 : Inport
  1-D Lookup Table : Lookup_n-D  NumberOfTableDimensions=1  BreakpointsSpecification=Even spacing  BreakpointsForDimension1=0:length(txDataOut)-1  BreakpointsForDimension1FirstPoint=0  Table=fi(DataLUT,1,18,16)  TableDataTypeStr=Inherit: Inherit from 'Table data'  InterpMethod=Flat  InternalRulePriority=Speed  OutDataTypeStr=fixdt(1, 18, 16)  RndMeth=Simplest
  1-D Lookup Table_pd1 : Delay  DelayLength=1
  Out1 : Outport
  wires:
  In1/1 -> 1-D Lookup Table/1
  1-D Lookup Table_pd1/1 -> Out1/1
  1-D Lookup Table/1 -> 1-D Lookup Table_pd1/1

== system gm_soc_dvbs2_fpga/DVBS2/DVBS2 TxRx/LUT Based Tx/Subsystem1/Subsystem4/txLUT4/1-D Lookup Table ==
  In1 : Inport
  1-D Lookup Table : Lookup_n-D  NumberOfTableDimensions=1  BreakpointsSpecification=Even spacing  BreakpointsForDimension1=0:length(txDataOut)-1  BreakpointsForDimension1FirstPoint=0  Table=fi(DataLUT,1,18,16)  TableDataTypeStr=Inherit: Inherit from 'Table data'  InterpMethod=Flat  InternalRulePriority=Speed  OutDataTypeStr=fixdt(1, 18, 16)  RndMeth=Simplest
  1-D Lookup Table_pd1 : Delay  DelayLength=1
  Out1 : Outport
  wires:
  In1/1 -> 1-D Lookup Table/1
  1-D Lookup Table_pd1/1 -> Out1/1
  1-D Lookup Table/1 -> 1-D Lookup Table_pd1/1

== system gm_soc_dvbs2_fpga/DVBS2/DVBS2 TxRx/LUT Based Tx/Subsystem1/Subsystem4/txLUT5/1-D Lookup Table ==
  In1 : Inport
  1-D Lookup Table : Lookup_n-D  NumberOfTableDimensions=1  BreakpointsSpecification=Even spacing  BreakpointsForDimension1=0:length(txDataOut)-1  BreakpointsForDimension1FirstPoint=0  Table=fi(DataLUT,1,18,16)  TableDataTypeStr=Inherit: Inherit from 'Table data'  InterpMethod=Flat  InternalRulePriority=Speed  OutDataTypeStr=fixdt(1, 18, 16)  RndMeth=Simplest
  1-D Lookup Table_pd1 : Delay  DelayLength=1
  Out1 : Outport
  wires:
  In1/1 -> 1-D Lookup Table/1
  1-D Lookup Table/1 -> 1-D Lookup Table_pd1/1
  1-D Lookup Table_pd1/1 -> Out1/1

== system gm_soc_dvbs2_fpga/DVBS2/DVBS2 TxRx/LUT Based Tx/Subsystem1/Subsystem4/txLUT6/1-D Lookup Table ==
  In1 : Inport
  1-D Lookup Table : Lookup_n-D  NumberOfTableDimensions=1  BreakpointsSpecification=Even spacing  BreakpointsForDimension1=0:length(txDataOut)-1  BreakpointsForDimension1FirstPoint=0  Table=fi(DataLUT,1,18,16)  TableDataTypeStr=Inherit: Inherit from 'Table data'  InterpMethod=Flat  InternalRulePriority=Speed  OutDataTypeStr=fixdt(1, 18, 16)  RndMeth=Simplest
  1-D Lookup Table_pd1 : Delay  DelayLength=1
  Out1 : Outport
  wires:
  In1/1 -> 1-D Lookup Table/1
  1-D Lookup Table_pd1/1 -> Out1/1
  1-D Lookup Table/1 -> 1-D Lookup Table_pd1/1
